simulink model "computed_torque"  (R2020b)
settings: Solver=VariableStepAuto  StartTime=0.0  StopTime=time  RelTol=1e-3
values from neighbouring files (symbols this model uses):
  Ath = 0.5    [main.m]
  b = sym('b','real')    [Oss_par.m]    (also in main.m = 0.2)
  gravity = sym('gravity','real')    [Oss_par.m]    (also in main.m = 9.81)
  I = sym('I','real')    [Oss_par.m]    (also in main.m = 235.2)
  K = sym('K','real')    [Oss_par.m]    (also in main.m = 40.248)
  L = sym('L','real')    [Oss_par.m]    (also in dir_der.m = h * f; main.m = 2.1)
  m = sym('m','real')    [Oss_par.m]    (also in main.m = 160)
  R = sym('R','real')    [Oss_par.m]    (also in main.m = 0.6)
  selector = select(1)    [main.m]    (also in select.m = input('? '))
  wth = 0.2    [main.m]
settings Model: Creator=Tommaso  LastModifiedBy=Tommaso
settings DataIOCC: ReturnWorkspaceOutputs=off

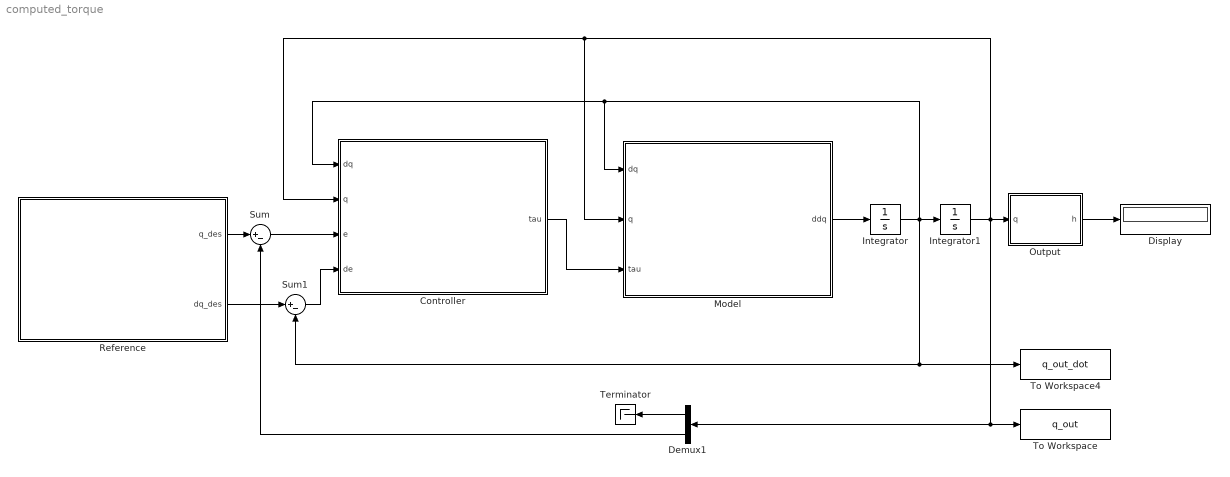
== system computed_torque ==
  Controller : MATLAB Function  TreatAsAtomicUnit=on
  Demux1 : Demux  Outputs=2
  Display : Display
  Integrator : Integrator  InitialCondition=[0; 0]
  Integrator1 : Integrator  InitialCondition=[0; pi/12]
  Model : MATLAB Function  TreatAsAtomicUnit=on
  Output : MATLAB Function  TreatAsAtomicUnit=on
  Reference : Subsystem
  Sum : Sum  Inputs=|+-
  Sum1 : Sum  Inputs=|+-
  Terminator : Terminator
  To Workspace : ToWorkspace  VariableName=q_out  SaveFormat=Timeseries  SampleTime=-1
  To Workspace4 : ToWorkspace  VariableName=q_out_dot  SaveFormat=Timeseries  SampleTime=-1
  wires:
  Output/1(h) -> Display/1
  Model/1(ddq) -> Integrator/1
  Integrator/1 -> Integrator1/1, Model/1(dq), Controller/1(dq), To Workspace4/1, Sum1/2
  Integrator1/1 -> Output/1(q), Model/2(q), Controller/2(q), To Workspace/1, Demux1/1
  Controller/1(tau) -> Model/3(tau)
  Sum/1 -> Controller/3(e)
  Sum1/1 -> Controller/4(de)
  Demux1/2 -> Sum/2
  Demux1/1 -> Terminator/1
  Reference/1(q_des) -> Sum/1
  Reference/2(dq_des) -> Sum1/1

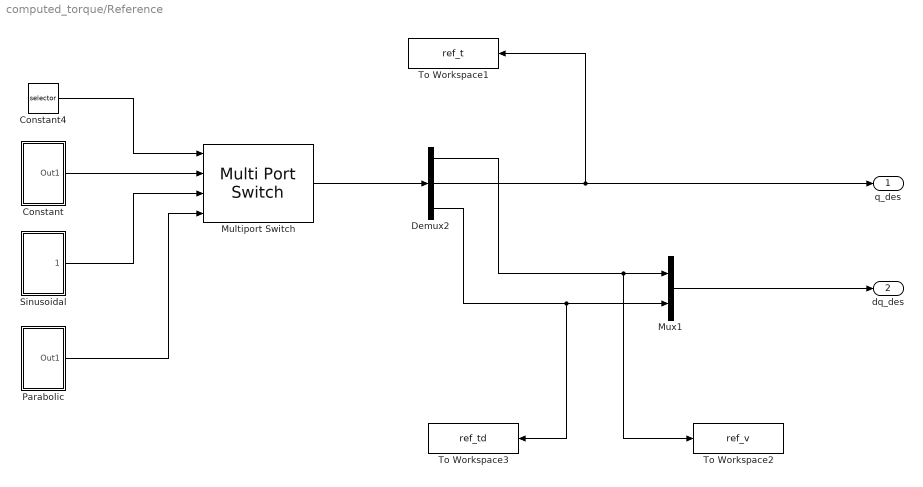
== system computed_torque/Reference ==
  Constant : Subsystem
  Constant4 : Constant  Value=selector
  Demux2 : Demux  Outputs=3
  Multiport Switch : MultiPortSwitch
  Mux1 : Mux  Inputs=2
  Parabolic : Subsystem
  Sinusoidal : Subsystem
  To Workspace1 : ToWorkspace  VariableName=ref_t  SaveFormat=Timeseries  SampleTime=-1
  To Workspace2 : ToWorkspace  VariableName=ref_v  SaveFormat=Timeseries  SampleTime=-1
  To Workspace3 : ToWorkspace  VariableName=ref_td  SaveFormat=Timeseries  SampleTime=-1
  q_des : Outport
  dq_des : Outport  Port=2
  wires:
  Demux2/1 -> To Workspace2/1, Mux1/1
  Demux2/3 -> To Workspace3/1, Mux1/2
  Demux2/2 -> To Workspace1/1, q_des/1
  Constant/1(Out1) -> Multiport Switch/2
  Parabolic/1(Out1) -> Multiport Switch/4
  Mux1/1 -> dq_des/1
  Constant4/1 -> Multiport Switch/1
  Multiport Switch/1 -> Demux2/1
  Sinusoidal/1(Outport) -> Multiport Switch/3

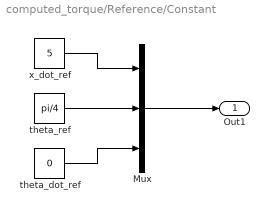
== system computed_torque/Reference/Constant ==
  Mux : Mux  Inputs=3
  theta_dot_ref : Constant  Value=0
  theta_ref : Constant  Value=pi/4
  x_dot_ref : Constant  Value=5
  Out1 : Outport
  wires:
  theta_ref/1 -> Mux/2
  theta_dot_ref/1 -> Mux/3
  Mux/1 -> Out1/1
  x_dot_ref/1 -> Mux/1

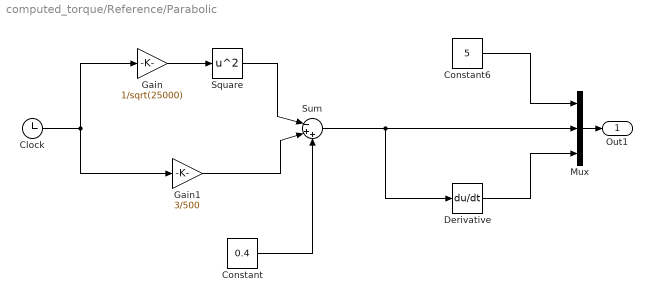
== system computed_torque/Reference/Parabolic ==
  Clock : Clock
  Constant : Constant  Value=0.4
  Constant6 : Constant  Value=5
  Derivative : Derivative
  Gain : Gain  Gain=1/sqrt(25000)
  Gain1 : Gain  Gain=3/500
  Mux : Mux  Inputs=3
  Square : Math  Operator=square  SaturateOnIntegerOverflow=on
  Sum : Sum  Inputs=|-++
  Out1 : Outport
  wires:
  Mux/1 -> Out1/1
  Gain/1 -> Square/1
  Derivative/1 -> Mux/3
  Square/1 -> Sum/1
  Sum/1 -> Mux/2, Derivative/1
  Gain1/1 -> Sum/2
  Clock/1 -> Gain1/1, Gain/1
  Constant6/1 -> Mux/1
  Constant/1 -> Sum/3

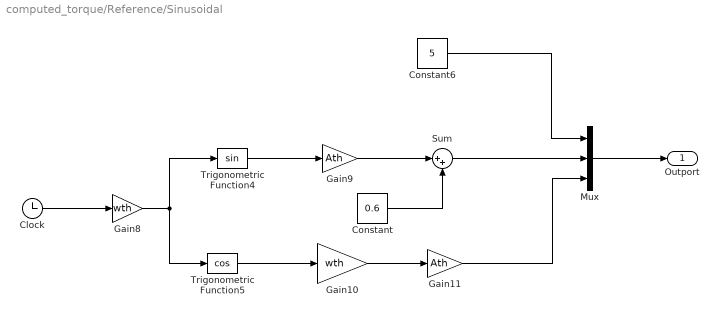
== system computed_torque/Reference/Sinusoidal ==
  Clock : Clock
  Constant : Constant  Value=0.6
  Constant6 : Constant  Value=5
  Gain10 : Gain  Gain=wth
  Gain11 : Gain  Gain=Ath
  Gain8 : Gain  Gain=wth
  Gain9 : Gain  Gain=Ath
  Mux : Mux  Inputs=3
  Sum : Sum  Inputs=|++
  Trigonometric Function4 : Trigonometry
  Trigonometric Function5 : Trigonometry  Operator=cos
  Outport : Outport
  wires:
  Gain11/1 -> Mux/3
  Trigonometric Function5/1 -> Gain10/1
  Gain10/1 -> Gain11/1
  Gain8/1 -> Trigonometric Function4/1, Trigonometric Function5/1
  Constant/1 -> Sum/2
  Clock/1 -> Gain8/1
  Gain9/1 -> Sum/1
  Mux/1 -> Outport/1
  Trigonometric Function4/1 -> Gain9/1
  Sum/1 -> Mux/2
  Constant6/1 -> Mux/1

== matlab function computed_torque/Output ==
  data: q input; h output; L parameter
function h = output(q, L)

% Output
h = L*sin(q(2));

== matlab function computed_torque/Model ==
  data: m parameter; R parameter; gravity parameter; L parameter; dq input; K parameter; b parameter; I parameter; q input; tau input; ddq output
function ddq = model(m, R, gravity, L, dq, K, b, I, q, tau)

% Configuration variables
theta = q(2);
x_dot = dq(1);

% Inertial matrix (2x2)
M = [m*R 0; 0 I];

% Damping matrix (2x2)
C = [(R/2)*K*(1+sin(theta))*x_dot 0; -(L/4)*K*(1+sin(theta))*x_dot*sin(theta) b];

% Potential vector (2x1)
G = [0; m*gravity*(L/2)*cos(theta)];

% Dynamic equation
ddq = M^(-1)*(tau - C*dq - G);

== matlab function computed_torque/Controller ==
  data: dq input; q input; tau output; m parameter; R parameter; gravity parameter; L parameter; K parameter; b parameter; I parameter; e input; de input
function tau = controller(dq, q, m, R, gravity, L, K, b, I, e, de)

% Configurations variables
theta = q(2);
x_dot = dq(1);

% Gains
Kv = 200*eye(2);
Kp = 800*eye(2);
% Inertial matrix (2x2)
M = [m*R 0; 0 I];

% Damping matrix (2x2)
C = [(R/2)*K*(1+sin(theta))*x_dot 0; -(L/4)*K*(1+sin(theta))*x_dot*sin(theta) b];

% Potential vector (2x1)
G = [0; m*gravity*(L/2)*cos(theta)];

% Errors
E = [0; e];
dE = de;

% Control output (2x1)
tau = (Kv*dE + Kp*E) + C*dq + G;

% tau moltiplicato per M, Kv = 20 e Kp = 80
